simulink model "test_pi_av_formation_event_gazebodirected23a"  (R2023a)
settings: Solver=FixedStepAuto  StartTime=0.0  StopTime=inf  RelTol=1e-3
undefined symbols (not defined in the file or in its folder): angular, DiscIntNeverNeededParam, linear
libraries: ros2lib x28, simulink x8, robotcorelib x8
(part 4 of 4)

== matlab function test_pi_av_formation_event_gazebodirected23a/Translational Control1/Flocking1/MATLAB Function2 ==
  data: ui_prev input; xi input; yi input; zi input; ui_gamma output; xr1 input; yr1 input; zr1 input; xr2 input; yr2 input; zr2 input; xr3 input; yr3 input; zr3 input; iep input size=3; norm_ex input; norm_ey input; norm_ez input; ep output size=3; K_cts input

function [ui_gamma, ep] = naviFeedback(ui_prev, xi, yi, zi, xr1, yr1, zr1, xr2, yr2, zr2, xr3, yr3, zr3, iep, norm_ex, norm_ey, norm_ez, K_cts)
    
    Kpxy = K_cts(1); Kixy = K_cts(2);
    xmin_xy = K_cts(3); xmax_xy = K_cts(4);
    Kpz = K_cts(5); Kiz = K_cts(6);
    xmin_z = K_cts(7); xmax_z = K_cts(8);

    %Sepration control
    ui_xprev = ui_prev(1); ui_yprev = ui_prev(2); ui_zprev = ui_prev(3);

%Errors
    e_x = (xi - xr1 + 0.55) + (xi - xr2) + (xi - xr3 + 1.1);

    e_y = (yi - yr1 + 0.55) + (yi - yr2 + 1.1) + (yi - yr3 + 1.1);

    e_z = (zi - zr1 + 0.55) + (zi - zr2 + 1.1) + (zi - zr3);
       
    ep = [e_x;e_y;e_z];

    if  norm_ex >= 0
        ui_gammax = (-1)* satFcn_esc(Kpxy*e_x, xmin_xy, xmax_xy) + (-1)* satFcn_esc(Kixy*iep(1), xmin_xy, xmax_xy);
    else
        ui_gammax = ui_xprev;
    end

    if  norm_ey >= 0
        ui_gammay = (-1)* satFcn_esc(Kpxy*e_y, xmin_xy, xmax_xy) + (-1)* satFcn_esc(Kixy*iep(1), xmin_xy, xmax_xy);
    else
        ui_gammay = ui_yprev;
    end

    if  norm_ez >= 0
        ui_gammaz = (-1)* satFcn_esc(Kpz*e_z, xmin_z, xmax_z) + (-1)*satFcn_esc(Kiz*iep(3), xmin_z, xmax_z);
    else
        ui_gammaz = ui_zprev;
    end
    

    ui_gamma = [ui_gammax;ui_gammay;ui_gammaz];
    
end

== matlab function test_pi_av_formation_event_gazebodirected23a/Translational Control2/Flocking1/MATLAB Function5 ==
  data: dot_hat_q output; L input; q input; q_hat input; eta1 input; eta2 input; u input; dot_eta output; ddot_eta output
function [dot_hat_q, dot_eta, ddot_eta] = fcn(L, q, q_hat, eta1, eta2, u)

%%separation gains vectors
l2 = [L(1) L(2) L(3)];
l1 = [L(4) L(5) L(6)];
l0 = [L(7) L(8) L(9)];

L_2 = diag(l2);
L_1 = diag(l1);
L_0 = diag(l0);

dot_hat_q = q_est(u, eta1, L_2, q, q_hat);

dot_eta = dot_eta_one(eta2, L_1, q, q_hat);

ddot_eta = dot_eta_two(L_0, q, q_hat);

== matlab function test_pi_av_formation_event_gazebodirected23a/Translational Control3/Flocking1/MATLAB Function5 ==
  data: dot_hat_q output; L input; q input; q_hat input; eta1 input; eta2 input; u input; dot_eta output; ddot_eta output
function [dot_hat_q, dot_eta, ddot_eta] = fcn(L, q, q_hat, eta1, eta2, u)

%%separation gains vectors
l2 = [L(1) L(2) L(3)];
l1 = [L(4) L(5) L(6)];
l0 = [L(7) L(8) L(9)];

L_2 = diag(l2);
L_1 = diag(l1);
L_0 = diag(l0);

dot_hat_q = q_est(u, eta1, L_2, q, q_hat);

dot_eta = dot_eta_one(eta2, L_1, q, q_hat);

ddot_eta = dot_eta_two(L_0, q, q_hat);

== matlab function test_pi_av_formation_event_gazebodirected23a/Translational Control5/Flocking1/MATLAB Function3 ==
  data: ui_prev input; xi input; yi input; zi input; ui_gamma output; xr1 input; yr1 input; zr1 input; xr2 input; yr2 input; zr2 input; iep input size=3; norm_ex input; norm_ey input; norm_ez input; ep output size=3; K_cts input

function [ui_gamma, ep] = naviFeedback(ui_prev, xi, yi, zi, xr1, yr1, zr1, xr2, yr2, zr2, iep, norm_ex, norm_ey, norm_ez, K_cts)
    
    Kpxy = K_cts(1); Kixy = K_cts(2);
    xmin_xy = K_cts(3); xmax_xy = K_cts(4);
    Kpz = K_cts(5); Kiz = K_cts(6);
    xmin_z = K_cts(7); xmax_z = K_cts(8);

    %Sepration control
    ui_xprev = ui_prev(1); ui_yprev = ui_prev(2); ui_zprev = ui_prev(3);

%Errors
    e_x = (xi - xr1 + 0.55) + (xi - xr2 + 1.1);

    e_y = (yi - yr1 + 0.55) + (yi - yr2 + 1.1);

    e_z = (zi - zr1 - 1.1) + (zi - zr2 - 1.1);
       
    ep = [e_x;e_y;e_z];

    if  norm_ex >= 0
        ui_gammax = (-1)* satFcn_esc(Kpxy*e_x, xmin_xy, xmax_xy) + (-1)* satFcn_esc(Kixy*iep(1), xmin_xy, xmax_xy);
    else
        ui_gammax = ui_xprev;
    end

    if  norm_ey >= 0
        ui_gammay = (-1)* satFcn_esc(Kpxy*e_y, xmin_xy, xmax_xy) + (-1)* satFcn_esc(Kixy*iep(1), xmin_xy, xmax_xy);
    else
        ui_gammay = ui_yprev;
    end

    if  norm_ez >= 0
        ui_gammaz = (-1)* satFcn_esc(Kpz*e_z, xmin_z, xmax_z) + (-1)*satFcn_esc(Kiz*iep(3), xmin_z, xmax_z);
    else
        ui_gammaz = ui_zprev;
    end
    

    ui_gamma = [ui_gammax;ui_gammay;ui_gammaz];
    
end

== matlab function test_pi_av_formation_event_gazebodirected23a/Translational Control5/Flocking1/MATLAB Function ==
  data: xi input; yi input; zi input; phiAlpha output; xj input; yj input; zj input; xk input; yk input; zk input; xl input; yl input; zl input; xm input; ym input; zm input; xn input; yn input; zn input; xo input; yo input; zo input; xp input; yp input; zp input; params input

function phiAlpha  = phiAlphaFcn(xi, yi, zi, xj, yj, zj, xk, yk, zk, xl, yl, zl, xm, ym, zm, xn, yn, zn, xo, yo, zo, xp, yp, zp, params)
    
    % Flocking parameters
    epsilon = params(1); a = params(2); b = params(3); c = params(4); d = params(5); h = params(6);

    e = abs(a - b) / sqrt(4*a*b) ;

    cAlpha = sigmaNormFun(c, epsilon) ;
    dAlpha = sigmaNormFun(d, epsilon) ;

    %%
    Pi = [xi;yi;zi] ;

    Pj = [xj;yj;zj] ;
    Pk = [xk;yk;zk] ;
    Pl = [xl;yl;zl] ;
    Pm = [xm;ym;zm] ;
    Pn = [xn;yn;zn] ;
    Po = [xo;yo;zo] ;
    Pp = [xp;yp;zp] ;

    %%
    sigmaNormj = sigmaNormFun(Pj - Pi, epsilon) ;
    nij = gradSigmaFun(Pj - Pi, epsilon) ;
    
    sigmaNormk = sigmaNormFun(Pk - Pi, epsilon) ;
    nik = gradSigmaFun(Pk - Pi, epsilon) ;

    sigmaNorml = sigmaNormFun(Pl - Pi, epsilon) ;
    nil = gradSigmaFun(Pl - Pi, epsilon) ;

    sigmaNormm = sigmaNormFun(Pm - Pi, epsilon) ;
    nim = gradSigmaFun(Pm - Pi, epsilon) ;

    sigmaNormn = sigmaNormFun(Pn - Pi, epsilon) ;
    nin = gradSigmaFun(Pn - Pi, epsilon) ;

    sigmaNormo = sigmaNormFun(Po - Pi, epsilon) ;
    nio = gradSigmaFun(Po - Pi, epsilon) ;

    sigmaNormp = sigmaNormFun(Pp - Pi, epsilon) ;
    nip = gradSigmaFun(Pp - Pi, epsilon) ;

    %%
    sigma1j = sigma1Fun(sigmaNormj - dAlpha + e) ;
    sigma1k = sigma1Fun(sigmaNormk - dAlpha + e) ;
    sigma1l = sigma1Fun(sigmaNorml - dAlpha + e) ;
    sigma1m = sigma1Fun(sigmaNormm - dAlpha + e) ;
    sigma1n = sigma1Fun(sigmaNormn - dAlpha + e) ;
    sigma1o = sigma1Fun(sigmaNormo - dAlpha + e) ;
    sigma1p = sigma1Fun(sigmaNormp - dAlpha + e) ;
            
    %% Position
    phiAlphaj = 0.5 * bumpFcn(sigmaNormj/cAlpha,h) * ((a+b)*sigma1j + (a-b)) ;
    phiAlphanij = phiAlphaj.* nij ;
    
    phiAlphak = 0.5 * bumpFcn(sigmaNormk/cAlpha,h) * ((a+b)*sigma1k + (a-b)) ;
    phiAlphanik = phiAlphak.* nik ;

    phiAlphal = 0.5 * bumpFcn(sigmaNorml/cAlpha,h) * ((a+b)*sigma1l + (a-b)) ;
    phiAlphanil = phiAlphal.* nil ;

    phiAlpham = 0.5 * bumpFcn(sigmaNormm/cAlpha,h) * ((a+b)*sigma1m + (a-b)) ;
    phiAlphanim = phiAlpham.* nim ;

    phiAlphan = 0.5 * bumpFcn(sigmaNormn/cAlpha,h) * ((a+b)*sigma1n + (a-b)) ;
    phiAlphanin = phiAlphan.* nin ;

    phiAlphao = 0.5 * bumpFcn(sigmaNormo/cAlpha,h) * ((a+b)*sigma1o + (a-b)) ;
    phiAlphanio = phiAlphao.* nio ;

    phiAlphap = 0.5 * bumpFcn(sigmaNormp/cAlpha,h) * ((a+b)*sigma1p + (a-b)) ;
    phiAlphanip = phiAlphap.* nip ;


    phiAlpha = phiAlphanij + phiAlphanik + phiAlphanil + phiAlphanim  + phiAlphanin + phiAlphanio + phiAlphanip;

    
end

== matlab function test_pi_av_formation_event_gazebodirected23a/Translational Control5/Flocking1/MATLAB Function1 ==
  data: eta input; phiAlpha input; phiAlpha_int input; ui_gamma input; yaw input; ieyaw input; Ui_pos output size=3; ui_yaw output; KP input; eyaw2 output size=1; eyaw1 input; eyaw2 input; eyaw3 input; eyaw4 input; eyaw6 input; eyaw7 input; eyaw8 input

function [Ui_pos, ui_yaw, eyaw2]  = ctrlLaw(eta, phiAlpha, phiAlpha_int, ui_gamma, yaw, ieyaw, KP, eyaw1, eyaw2, eyaw3, eyaw4, eyaw6, eyaw7, eyaw8)  %, phiBetak, bikobs, phiBetanei, bikve
    
    % Control gains and parameters
    Kx = KP(1); Ky = KP(2); Kz = KP(3);
    Kix = KP(4); Kiy = KP(5); Kiz = KP(6);
    Kyaw = KP(7); Kdyaw = KP(8); Kiyaw = KP(9);
    offset = KP(10);

    eyaw = 0 - yaw(1);
    deyaw = 0 - yaw(2);

    ui_yaw = Kyaw*eyaw + Kdyaw*deyaw + Kiyaw*ieyaw;
    hz_dot = Kz * phiAlpha(3,1) + Kiz * phiAlpha_int(3,1) + ui_gamma(3,1) - eta(3,1);  
    
    if eyaw < offset && eyaw > -offset && eyaw1 < offset && eyaw1 > -offset && eyaw2 < offset && eyaw2 > -offset && eyaw3 < offset && eyaw3 > -offset && eyaw4 < offset && eyaw4 > -offset && eyaw6 < offset && eyaw6 > -offset && eyaw7 < offset && eyaw7 > -offset && eyaw8 < offset && eyaw8 > -offset
        hx_dot = Kx * phiAlpha(1,1) + Kix * phiAlpha_int(1,1) + ui_gamma(1,1) - eta(1,1);  
        hy_dot = Ky * phiAlpha(2,1) + Kiy * phiAlpha_int(2,1) + ui_gamma(2,1) - eta(2,1);  
    else
        hx_dot = 0;
        hy_dot = 0;
    end

    Ui_pos = [hx_dot; hy_dot; hz_dot] ;
    

end

== matlab function test_pi_av_formation_event_gazebodirected23a/Translational Control6/Flocking1/MATLAB Function3 ==
  data: ui_prev input; xi input; yi input; zi input; ui_gamma output; xr1 input; yr1 input; zr1 input; xr2 input; yr2 input; zr2 input; xr3 input; yr3 input; zr3 input; iep input size=3; norm_ex input; norm_ey input; norm_ez input; ep output size=3; K_cts input

function [ui_gamma, ep] = naviFeedback(ui_prev, xi, yi, zi, xr1, yr1, zr1, xr2, yr2, zr2, xr3, yr3, zr3, iep, norm_ex, norm_ey, norm_ez, K_cts)
    
    Kpxy = K_cts(1); Kixy = K_cts(2);
    xmin_xy = K_cts(3); xmax_xy = K_cts(4);
    Kpz = K_cts(5); Kiz = K_cts(6);
    xmin_z = K_cts(7); xmax_z = K_cts(8);

    %Sepration control
    ui_xprev = ui_prev(1); ui_yprev = ui_prev(2); ui_zprev = ui_prev(3);

%Errors
    e_x = (xi - xr1 - 0.55) + (xi - xr2) + (xi - xr3 - 1.1);

    e_y = (yi - yr1 + 0.55) + (yi - yr2 + 1.1) + (yi - yr3);

    e_z = (zi - zr1 - 0.55) + (zi - zr2 - 1.1) + (zi - zr3);
       
    ep = [e_x;e_y;e_z];

    if  norm_ex >= 0
        ui_gammax = (-1)* satFcn_esc(Kpxy*e_x, xmin_xy, xmax_xy) + (-1)* satFcn_esc(Kixy*iep(1), xmin_xy, xmax_xy);
    else
        ui_gammax = ui_xprev;
    end

    if  norm_ey >= 0
        ui_gammay = (-1)* satFcn_esc(Kpxy*e_y, xmin_xy, xmax_xy) + (-1)* satFcn_esc(Kixy*iep(1), xmin_xy, xmax_xy);
    else
        ui_gammay = ui_yprev;
    end

    if  norm_ez >= 0
        ui_gammaz = (-1)* satFcn_esc(Kpz*e_z, xmin_z, xmax_z) + (-1)*satFcn_esc(Kiz*iep(3), xmin_z, xmax_z);
    else
        ui_gammaz = ui_zprev;
    end
    

    ui_gamma = [ui_gammax;ui_gammay;ui_gammaz];
    
end

== matlab function test_pi_av_formation_event_gazebodirected23a/Translational Control5/Flocking1/MATLAB Function5 ==
  data: dot_hat_q output; L input; q input; q_hat input; eta1 input; eta2 input; u input; dot_eta output; ddot_eta output
function [dot_hat_q, dot_eta, ddot_eta] = fcn(L, q, q_hat, eta1, eta2, u)

%%separation gains vectors
l2 = [L(1) L(2) L(3)];
l1 = [L(4) L(5) L(6)];
l0 = [L(7) L(8) L(9)];

L_2 = diag(l2);
L_1 = diag(l1);
L_0 = diag(l0);

dot_hat_q = q_est(u, eta1, L_2, q, q_hat);

dot_eta = dot_eta_one(eta2, L_1, q, q_hat);

ddot_eta = dot_eta_two(L_0, q, q_hat);

== matlab function test_pi_av_formation_event_gazebodirected23a/Translational Control7/Flocking1/MATLAB Function ==
  data: xi input; yi input; zi input; phiAlpha output; xj input; yj input; zj input; xk input; yk input; zk input; xl input; yl input; zl input; xm input; ym input; zm input; xn input; yn input; zn input; xo input; yo input; zo input; xp input; yp input; zp input; params input

function phiAlpha  = phiAlphaFcn(xi, yi, zi, xj, yj, zj, xk, yk, zk, xl, yl, zl, xm, ym, zm, xn, yn, zn, xo, yo, zo, xp, yp, zp, params)
    
    % Flocking parameters
    epsilon = params(1); a = params(2); b = params(3); c = params(4); d = params(5); h = params(6);

    e = abs(a - b) / sqrt(4*a*b) ;

    cAlpha = sigmaNormFun(c, epsilon) ;
    dAlpha = sigmaNormFun(d, epsilon) ;

    %%
    Pi = [xi;yi;zi] ;

    Pj = [xj;yj;zj] ;
    Pk = [xk;yk;zk] ;
    Pl = [xl;yl;zl] ;
    Pm = [xm;ym;zm] ;
    Pn = [xn;yn;zn] ;
    Po = [xo;yo;zo] ;
    Pp = [xp;yp;zp] ;

    %%
    sigmaNormj = sigmaNormFun(Pj - Pi, epsilon) ;
    nij = gradSigmaFun(Pj - Pi, epsilon) ;
    
    sigmaNormk = sigmaNormFun(Pk - Pi, epsilon) ;
    nik = gradSigmaFun(Pk - Pi, epsilon) ;

    sigmaNorml = sigmaNormFun(Pl - Pi, epsilon) ;
    nil = gradSigmaFun(Pl - Pi, epsilon) ;

    sigmaNormm = sigmaNormFun(Pm - Pi, epsilon) ;
    nim = gradSigmaFun(Pm - Pi, epsilon) ;

    sigmaNormn = sigmaNormFun(Pn - Pi, epsilon) ;
    nin = gradSigmaFun(Pn - Pi, epsilon) ;

    sigmaNormo = sigmaNormFun(Po - Pi, epsilon) ;
    nio = gradSigmaFun(Po - Pi, epsilon) ;

    sigmaNormp = sigmaNormFun(Pp - Pi, epsilon) ;
    nip = gradSigmaFun(Pp - Pi, epsilon) ;

    %%
    sigma1j = sigma1Fun(sigmaNormj - dAlpha + e) ;
    sigma1k = sigma1Fun(sigmaNormk - dAlpha + e) ;
    sigma1l = sigma1Fun(sigmaNorml - dAlpha + e) ;
    sigma1m = sigma1Fun(sigmaNormm - dAlpha + e) ;
    sigma1n = sigma1Fun(sigmaNormn - dAlpha + e) ;
    sigma1o = sigma1Fun(sigmaNormo - dAlpha + e) ;
    sigma1p = sigma1Fun(sigmaNormp - dAlpha + e) ;
            
    %% Position
    phiAlphaj = 0.5 * bumpFcn(sigmaNormj/cAlpha,h) * ((a+b)*sigma1j + (a-b)) ;
    phiAlphanij = phiAlphaj.* nij ;
    
    phiAlphak = 0.5 * bumpFcn(sigmaNormk/cAlpha,h) * ((a+b)*sigma1k + (a-b)) ;
    phiAlphanik = phiAlphak.* nik ;

    phiAlphal = 0.5 * bumpFcn(sigmaNorml/cAlpha,h) * ((a+b)*sigma1l + (a-b)) ;
    phiAlphanil = phiAlphal.* nil ;

    phiAlpham = 0.5 * bumpFcn(sigmaNormm/cAlpha,h) * ((a+b)*sigma1m + (a-b)) ;
    phiAlphanim = phiAlpham.* nim ;

    phiAlphan = 0.5 * bumpFcn(sigmaNormn/cAlpha,h) * ((a+b)*sigma1n + (a-b)) ;
    phiAlphanin = phiAlphan.* nin ;

    phiAlphao = 0.5 * bumpFcn(sigmaNormo/cAlpha,h) * ((a+b)*sigma1o + (a-b)) ;
    phiAlphanio = phiAlphao.* nio ;

    phiAlphap = 0.5 * bumpFcn(sigmaNormp/cAlpha,h) * ((a+b)*sigma1p + (a-b)) ;
    phiAlphanip = phiAlphap.* nip ;


    phiAlpha = phiAlphanij + phiAlphanik + phiAlphanil + phiAlphanim  + phiAlphanin + phiAlphanio + phiAlphanip;

    
end

== matlab function test_pi_av_formation_event_gazebodirected23a/Translational Control7/Flocking1/MATLAB Function1 ==
  data: eta input; phiAlpha input; phiAlpha_int input; ui_gamma input; yaw input; ieyaw input; Ui_pos output size=3; ui_yaw output; KP input; eyaw2 output size=1; eyaw1 input; eyaw2 input; eyaw3 input; eyaw4 input; eyaw5 input; eyaw6 input; eyaw8 input

function [Ui_pos, ui_yaw, eyaw2]  = ctrlLaw(eta, phiAlpha, phiAlpha_int, ui_gamma, yaw, ieyaw, KP, eyaw1, eyaw2, eyaw3, eyaw4, eyaw5, eyaw6, eyaw8)  %, phiBetak, bikobs, phiBetanei, bikve
    
    % Control gains and parameters
    Kx = KP(1); Ky = KP(2); Kz = KP(3);
    Kix = KP(4); Kiy = KP(5); Kiz = KP(6);
    Kyaw = KP(7); Kdyaw = KP(8); Kiyaw = KP(9);
    offset = KP(10);

    eyaw = 0 - yaw(1);
    deyaw = 0 - yaw(2);

    ui_yaw = Kyaw*eyaw + Kdyaw*deyaw + Kiyaw*ieyaw;
    hz_dot = Kz * phiAlpha(3,1) + Kiz * phiAlpha_int(3,1) + ui_gamma(3,1) - eta(3,1);  
    
    if eyaw < offset && eyaw > -offset && eyaw1 < offset && eyaw1 > -offset && eyaw2 < offset && eyaw2 > -offset && eyaw3 < offset && eyaw3 > -offset && eyaw4 < offset && eyaw4 > -offset && eyaw5 < offset && eyaw5 > -offset && eyaw6 < offset && eyaw6 > -offset && eyaw8 < offset && eyaw8 > -offset
        hx_dot = Kx * phiAlpha(1,1) + Kix * phiAlpha_int(1,1) + ui_gamma(1,1) - eta(1,1);  
        hy_dot = Ky * phiAlpha(2,1) + Kiy * phiAlpha_int(2,1) + ui_gamma(2,1) - eta(2,1);  
    else
        hx_dot = 0;
        hy_dot = 0;
    end

    Ui_pos = [hx_dot; hy_dot; hz_dot] ;
    

end

== matlab function test_pi_av_formation_event_gazebodirected23a/Translational Control8/Flocking1/MATLAB Function3 ==
  data: ui_prev input; xi input; yi input; zi input; ui_gamma output; xr1 input; yr1 input; zr1 input; xr2 input; yr2 input; zr2 input; xr3 input; yr3 input; zr3 input; iep input size=3; norm_ex input; norm_ey input; norm_ez input; ep output size=3; K_cts input

function [ui_gamma, ep] = naviFeedback(ui_prev, xi, yi, zi, xr1, yr1, zr1, xr2, yr2, zr2, xr3, yr3, zr3, iep, norm_ex, norm_ey, norm_ez, K_cts)
    
    Kpxy = K_cts(1); Kixy = K_cts(2);
    xmin_xy = K_cts(3); xmax_xy = K_cts(4);
    Kpz = K_cts(5); Kiz = K_cts(6);
    xmin_z = K_cts(7); xmax_z = K_cts(8);

    %Sepration control
    ui_xprev = ui_prev(1); ui_yprev = ui_prev(2); ui_zprev = ui_prev(3);

%Errors
    e_x = (xi - xr1 + 0.55) + (xi - xr2)  + (xi - xr3 + 1.1);

    e_y = (yi - yr1 - 0.55) + (yi - yr2 - 1.1) + (yi - yr3);

    e_z = (zi - zr1 - 0.55) + (zi - zr2 - 1.1) + (zi - zr3 - 1.1);
       
    ep = [e_x;e_y;e_z];

    if  norm_ex >= 0
        ui_gammax = (-1)* satFcn_esc(Kpxy*e_x, xmin_xy, xmax_xy) + (-1)* satFcn_esc(Kixy*iep(1), xmin_xy, xmax_xy);
    else
        ui_gammax = ui_xprev;
    end

    if  norm_ey >= 0
        ui_gammay = (-1)* satFcn_esc(Kpxy*e_y, xmin_xy, xmax_xy) + (-1)* satFcn_esc(Kixy*iep(1), xmin_xy, xmax_xy);
    else
        ui_gammay = ui_yprev;
    end

    if  norm_ez >= 0
        ui_gammaz = (-1)* satFcn_esc(Kpz*e_z, xmin_z, xmax_z) + (-1)*satFcn_esc(Kiz*iep(3), xmin_z, xmax_z);
    else
        ui_gammaz = ui_zprev;
    end
    

    ui_gamma = [ui_gammax;ui_gammay;ui_gammaz];
    
end

== matlab function test_pi_av_formation_event_gazebodirected23a/Translational Control1/Flocking1/MATLAB Function5 ==
  data: dot_hat_q output; L input; q input; q_hat input; eta1 input; eta2 input; u input; dot_eta output; ddot_eta output
function [dot_hat_q, dot_eta, ddot_eta] = fcn(L, q, q_hat, eta1, eta2, u)

%%separation gains vectors
l2 = [L(1) L(2) L(3)];
l1 = [L(4) L(5) L(6)];
l0 = [L(7) L(8) L(9)];

L_2 = diag(l2);
L_1 = diag(l1);
L_0 = diag(l0);

dot_hat_q = q_est(u, eta1, L_2, q, q_hat);

dot_eta = dot_eta_one(eta2, L_1, q, q_hat);

ddot_eta = dot_eta_two(L_0, q, q_hat);

== matlab function test_pi_av_formation_event_gazebodirected23a/Translational Control7/Flocking1/MATLAB Function5 ==
  data: dot_hat_q output; L input; q input; q_hat input; eta1 input; eta2 input; u input; dot_eta output; ddot_eta output
function [dot_hat_q, dot_eta, ddot_eta] = fcn(L, q, q_hat, eta1, eta2, u)

%%separation gains vectors
l2 = [L(1) L(2) L(3)];
l1 = [L(4) L(5) L(6)];
l0 = [L(7) L(8) L(9)];

L_2 = diag(l2);
L_1 = diag(l1);
L_0 = diag(l0);

dot_hat_q = q_est(u, eta1, L_2, q, q_hat);

dot_eta = dot_eta_one(eta2, L_1, q, q_hat);

ddot_eta = dot_eta_two(L_0, q, q_hat);

== matlab function test_pi_av_formation_event_gazebodirected23a/Translational Control8/Flocking1/MATLAB Function ==
  data: xi input; yi input; zi input; phiAlpha output; xj input; yj input; zj input; xk input; yk input; zk input; xl input; yl input; zl input; xm input; ym input; zm input; xn input; yn input; zn input; xo input; yo input; zo input; xp input; yp input; zp input; params input

function phiAlpha  = phiAlphaFcn(xi, yi, zi, xj, yj, zj, xk, yk, zk, xl, yl, zl, xm, ym, zm, xn, yn, zn, xo, yo, zo, xp, yp, zp, params)
    
    % Flocking parameters
    epsilon = params(1); a = params(2); b = params(3); c = params(4); d = params(5); h = params(6);

    e = abs(a - b) / sqrt(4*a*b) ;

    cAlpha = sigmaNormFun(c, epsilon) ;
    dAlpha = sigmaNormFun(d, epsilon) ;

    %%
    Pi = [xi;yi;zi] ;

    Pj = [xj;yj;zj] ;
    Pk = [xk;yk;zk] ;
    Pl = [xl;yl;zl] ;
    Pm = [xm;ym;zm] ;
    Pn = [xn;yn;zn] ;
    Po = [xo;yo;zo] ;
    Pp = [xp;yp;zp] ;

    %%
    sigmaNormj = sigmaNormFun(Pj - Pi, epsilon) ;
    nij = gradSigmaFun(Pj - Pi, epsilon) ;
    
    sigmaNormk = sigmaNormFun(Pk - Pi, epsilon) ;
    nik = gradSigmaFun(Pk - Pi, epsilon) ;

    sigmaNorml = sigmaNormFun(Pl - Pi, epsilon) ;
    nil = gradSigmaFun(Pl - Pi, epsilon) ;

    sigmaNormm = sigmaNormFun(Pm - Pi, epsilon) ;
    nim = gradSigmaFun(Pm - Pi, epsilon) ;

    sigmaNormn = sigmaNormFun(Pn - Pi, epsilon) ;
    nin = gradSigmaFun(Pn - Pi, epsilon) ;

    sigmaNormo = sigmaNormFun(Po - Pi, epsilon) ;
    nio = gradSigmaFun(Po - Pi, epsilon) ;

    sigmaNormp = sigmaNormFun(Pp - Pi, epsilon) ;
    nip = gradSigmaFun(Pp - Pi, epsilon) ;

    %%
    sigma1j = sigma1Fun(sigmaNormj - dAlpha + e) ;
    sigma1k = sigma1Fun(sigmaNormk - dAlpha + e) ;
    sigma1l = sigma1Fun(sigmaNorml - dAlpha + e) ;
    sigma1m = sigma1Fun(sigmaNormm - dAlpha + e) ;
    sigma1n = sigma1Fun(sigmaNormn - dAlpha + e) ;
    sigma1o = sigma1Fun(sigmaNormo - dAlpha + e) ;
    sigma1p = sigma1Fun(sigmaNormp - dAlpha + e) ;
            
    %% Position
    phiAlphaj = 0.5 * bumpFcn(sigmaNormj/cAlpha,h) * ((a+b)*sigma1j + (a-b)) ;
    phiAlphanij = phiAlphaj.* nij ;
    
    phiAlphak = 0.5 * bumpFcn(sigmaNormk/cAlpha,h) * ((a+b)*sigma1k + (a-b)) ;
    phiAlphanik = phiAlphak.* nik ;

    phiAlphal = 0.5 * bumpFcn(sigmaNorml/cAlpha,h) * ((a+b)*sigma1l + (a-b)) ;
    phiAlphanil = phiAlphal.* nil ;

    phiAlpham = 0.5 * bumpFcn(sigmaNormm/cAlpha,h) * ((a+b)*sigma1m + (a-b)) ;
    phiAlphanim = phiAlpham.* nim ;

    phiAlphan = 0.5 * bumpFcn(sigmaNormn/cAlpha,h) * ((a+b)*sigma1n + (a-b)) ;
    phiAlphanin = phiAlphan.* nin ;

    phiAlphao = 0.5 * bumpFcn(sigmaNormo/cAlpha,h) * ((a+b)*sigma1o + (a-b)) ;
    phiAlphanio = phiAlphao.* nio ;

    phiAlphap = 0.5 * bumpFcn(sigmaNormp/cAlpha,h) * ((a+b)*sigma1p + (a-b)) ;
    phiAlphanip = phiAlphap.* nip ;


    phiAlpha = phiAlphanij + phiAlphanik + phiAlphanil + phiAlphanim  + phiAlphanin + phiAlphanio + phiAlphanip;

    
end

== matlab function test_pi_av_formation_event_gazebodirected23a/Translational Control4/Flocking1/MATLAB Function5 ==
  data: dot_hat_q output; L input; q input; q_hat input; eta1 input; eta2 input; u input; dot_eta output; ddot_eta output
function [dot_hat_q, dot_eta, ddot_eta] = fcn(L, q, q_hat, eta1, eta2, u)

%%separation gains vectors
l2 = [L(1) L(2) L(3)];
l1 = [L(4) L(5) L(6)];
l0 = [L(7) L(8) L(9)];

L_2 = diag(l2);
L_1 = diag(l1);
L_0 = diag(l0);

dot_hat_q = q_est(u, eta1, L_2, q, q_hat);

dot_eta = dot_eta_one(eta2, L_1, q, q_hat);

ddot_eta = dot_eta_two(L_0, q, q_hat);

== matlab function test_pi_av_formation_event_gazebodirected23a/Translational Control8/Flocking1/MATLAB Function1 ==
  data: eta input; phiAlpha input; phiAlpha_int input; ui_gamma input; yaw input; ieyaw input; Ui_pos output size=3; ui_yaw output; KP input; eyaw2 output size=1; eyaw1 input; eyaw2 input; eyaw3 input; eyaw4 input; eyaw5 input; eyaw6 input; eyaw7 input

function [Ui_pos, ui_yaw, eyaw2]  = ctrlLaw(eta, phiAlpha, phiAlpha_int, ui_gamma, yaw, ieyaw, KP, eyaw1, eyaw2, eyaw3, eyaw4, eyaw5, eyaw6, eyaw7)  %, phiBetak, bikobs, phiBetanei, bikve
    
    % Control gains and parameters
    Kx = KP(1); Ky = KP(2); Kz = KP(3);
    Kix = KP(4); Kiy = KP(5); Kiz = KP(6);
    Kyaw = KP(7); Kdyaw = KP(8); Kiyaw = KP(9);
    offset = KP(10);

    eyaw = 0 - yaw(1);
    deyaw = 0 - yaw(2);

    ui_yaw = Kyaw*eyaw + Kdyaw*deyaw + Kiyaw*ieyaw;
    hz_dot = Kz * phiAlpha(3,1) + Kiz * phiAlpha_int(3,1) + ui_gamma(3,1) - eta(3,1);  
    
    if eyaw < offset && eyaw > -offset && eyaw1 < offset && eyaw1 > -offset && eyaw2 < offset && eyaw2 > -offset && eyaw3 < offset && eyaw3 > -offset && eyaw4 < offset && eyaw4 > -offset && eyaw5 < offset && eyaw5 > -offset && eyaw6 < offset && eyaw6 > -offset && eyaw7 < offset && eyaw7 > -offset
        hx_dot = Kx * phiAlpha(1,1) + Kix * phiAlpha_int(1,1) + ui_gamma(1,1) - eta(1,1);  
        hy_dot = Ky * phiAlpha(2,1) + Kiy * phiAlpha_int(2,1) + ui_gamma(2,1) - eta(2,1);  
    else
        hx_dot = 0;
        hy_dot = 0;
    end

    Ui_pos = [hx_dot; hy_dot; hz_dot] ;
    

end

== matlab function test_pi_av_formation_event_gazebodirected23a/Translational Control1/Flocking1/event_x2 ==
  data: e_1 output; e_2 output; e1 input; e2 input; e3 input; e_3 output; i1 output; i1 input; i2 input; i3 input; i2 output; i3 output
function [e_1,e_2, e_3, i1, i2, i3]  = fcn(e1, e2, e3, i1, i2, i3)

if e1 >= 0
    e_1 = 1;
    i1 = i1+1;
else 
    e_1 = 0;
    i1 = i1;
end

if e2 >= 0
    e_2 = 1;
    i2 = i2 + 1;
else 
    e_2 = 0;
    i2 = i2;
end

if e3 >= 0
    e_3 = 1;
    i3 = i3 + 1;
else 
    e_3 = 0;
    i3 = i3;
end

== matlab function test_pi_av_formation_event_gazebodirected23a/Translational Control8/Flocking1/MATLAB Function5 ==
  data: dot_hat_q output; L input; q input; q_hat input; eta1 input; eta2 input; u input; dot_eta output; ddot_eta output
function [dot_hat_q, dot_eta, ddot_eta] = fcn(L, q, q_hat, eta1, eta2, u)

%%separation gains vectors
l2 = [L(1) L(2) L(3)];
l1 = [L(4) L(5) L(6)];
l0 = [L(7) L(8) L(9)];

L_2 = diag(l2);
L_1 = diag(l1);
L_0 = diag(l0);

dot_hat_q = q_est(u, eta1, L_2, q, q_hat);

dot_eta = dot_eta_one(eta2, L_1, q, q_hat);

ddot_eta = dot_eta_two(L_0, q, q_hat);

== matlab function test_pi_av_formation_event_gazebodirected23a/MATLAB Function2 ==
  data: data input; y output
function y = fcn(data)

DATA = data(1:20);
d1 = awgn(double(DATA(1)), 33, 'measured');
d2 = awgn(double(DATA(2)), 33, 'measured');
d3 = awgn(double(DATA(3)), 33, 'measured');
d4 = awgn(double(DATA(4)), 33, 'measured');
d5 = awgn(double(DATA(5)), 33, 'measured');
d6 = awgn(double(DATA(6)), 33, 'measured');
d7 = awgn(double(DATA(7)), 33, 'measured');
y = [d1;d2;d3;d4;d5;d6;d7];

== matlab function test_pi_av_formation_event_gazebodirected23a/Subsystem1/MATLAB Function6 ==
  data: X1 input; X2 input; X3 input; X4 input; X5 input; X6 input; X7 input; d_meas input; xyz output
function xyz = fcn(X1, X2, X3, X4, X5, X6, X7, d_meas)

%% Extract data from vectors
states1 = X1(1:3);
x1 = states1(1);
y1 = states1(2);
z1 = states1(3);

states2 = X2(1:3);
x2 = states2(1);
y2 = states2(2);
z2 = states2(3);

states3 = X3(1:3);
x3 = states3(1);
y3 = states3(2);
z3 = states3(3);

states4 = X4(1:3);
x4 = states4(1);
y4 = states4(2);
z4 = states4(3);

states5 = X5(1:3);
x5 = states5(1);
y5 = states5(2);
z5 = states5(3);

states6 = X6(1:3);
x6 = states6(1);
y6 = states6(2);
z6 = states6(3);

states7 = X7(1:3);
x7 = states7(1);
y7 = states7(2);
z7 = states7(3);

r1 = d_meas(1);
r2 = d_meas(2);
r3 = d_meas(3);
r4 = d_meas(4);
r5 = d_meas(5);
r6 = d_meas(6);
r7 = d_meas(7);

xyz = multi_fun2(x1, y1, z1, r1, x2, y2, z2, r2, x3, y3, z3, r3, x4, y4, z4, r4, x5, y5, z5, r5, x6, y6, z6, r6, x7, y7, z7, r7);

== matlab function test_pi_av_formation_event_gazebodirected23a/Subsystem1/dist_AVT ==
  data: meas input; u_B input; dU output; dAVT output; avt_pars input
function [dU,dAVT]  = fcn(meas, u_B, avt_pars)

%Vector separation
d1 = meas(1);
d2 = meas(2);
d3 = meas(3);
d4 = meas(4);
d5 = meas(5);
d6 = meas(6);
d7 = meas(7);

avtpars = avt_pars(1:4);
inc = avtpars(1);
dec = avtpars(2);
min = avtpars(3);
max = avtpars(4);

%% memory variables
d_avt1 = u_B(1);
adjustment1 = u_B(2);
s_adjust1 = u_B(3);

d_avt2 = u_B(4);
adjustment2 = u_B(5);
s_adjust2 = u_B(6);

d_avt3 = u_B(7);
adjustment3 = u_B(8);
s_adjust3 = u_B(9);

d_avt4 = u_B(10);
adjustment4 = u_B(11);
s_adjust4 = u_B(12);

d_avt5 = u_B(13);
adjustment5 = u_B(14);
s_adjust5 = u_B(15);

d_avt6 = u_B(16);
adjustment6 = u_B(17);
s_adjust6 = u_B(18);

d_avt7 = u_B(19);
adjustment7 = u_B(20);
s_adjust7 = u_B(21);

%%
du1 = AVTfun(d_avt1, d1, adjustment1, s_adjust1, min, max, inc, dec);

du2 = AVTfun(d_avt2, d2, adjustment2, s_adjust2, min, max, inc, dec);

du3 = AVTfun(d_avt3, d3, adjustment3, s_adjust3, min, max, inc, dec);

du4 = AVTfun(d_avt4, d4, adjustment4, s_adjust4, min, max, inc, dec);

du5 = AVTfun(d_avt5, d5, adjustment5, s_adjust5, min, max, inc, dec);

du6 = AVTfun(d_avt6, d6, adjustment6, s_adjust6, min, max, inc, dec);

du7 = AVTfun(d_avt7, d7, adjustment7, s_adjust7, min, max, inc, dec);

dU = [du1;du2;du3;du4;du5;du6;du7];
dAVT = [du1(1);du2(1);du3(1);du4(1);du5(1);du6(1);du7(1)];

== matlab function test_pi_av_formation_event_gazebodirected23a/MATLAB Function3 ==
  data: data input; y output
function y = fcn(data)

DATA = data(1:20);
d1 = awgn(double(DATA(1)), 33, 'measured');
d2 = awgn(double(DATA(2)), 33, 'measured');
d3 = awgn(double(DATA(3)), 33, 'measured');
d4 = awgn(double(DATA(4)), 33, 'measured');
d5 = awgn(double(DATA(5)), 33, 'measured');
d6 = awgn(double(DATA(6)), 33, 'measured');
d7 = awgn(double(DATA(7)), 33, 'measured');
y = [d1;d2;d3;d4;d5;d6;d7];

== matlab function test_pi_av_formation_event_gazebodirected23a/Subsystem2/MATLAB Function6 ==
  data: X1 input; X2 input; X3 input; X4 input; X5 input; X6 input; X7 input; d_meas input; xyz output
function xyz = fcn(X1, X2, X3, X4, X5, X6, X7, d_meas)

%% Extract data from vectors
states1 = X1(1:3);
x1 = states1(1);
y1 = states1(2);
z1 = states1(3);

states2 = X2(1:3);
x2 = states2(1);
y2 = states2(2);
z2 = states2(3);

states3 = X3(1:3);
x3 = states3(1);
y3 = states3(2);
z3 = states3(3);

states4 = X4(1:3);
x4 = states4(1);
y4 = states4(2);
z4 = states4(3);

states5 = X5(1:3);
x5 = states5(1);
y5 = states5(2);
z5 = states5(3);

states6 = X6(1:3);
x6 = states6(1);
y6 = states6(2);
z6 = states6(3);

states7 = X7(1:3);
x7 = states7(1);
y7 = states7(2);
z7 = states7(3);

r1 = d_meas(1);
r2 = d_meas(2);
r3 = d_meas(3);
r4 = d_meas(4);
r5 = d_meas(5);
r6 = d_meas(6);
r7 = d_meas(7);

xyz = multi_fun2(x1, y1, z1, r1, x2, y2, z2, r2, x3, y3, z3, r3, x4, y4, z4, r4, x5, y5, z5, r5, x6, y6, z6, r6, x7, y7, z7, r7);

== matlab function test_pi_av_formation_event_gazebodirected23a/Subsystem2/dist_AVT ==
  data: meas input; u_B input; dU output; dAVT output; avt_pars input
function [dU,dAVT]  = fcn(meas, u_B, avt_pars)

%Vector separation
d1 = meas(1);
d2 = meas(2);
d3 = meas(3);
d4 = meas(4);
d5 = meas(5);
d6 = meas(6);
d7 = meas(7);

avtpars = avt_pars(1:4);
inc = avtpars(1);
dec = avtpars(2);
min = avtpars(3);
max = avtpars(4);

%% memory variables
d_avt1 = u_B(1);
adjustment1 = u_B(2);
s_adjust1 = u_B(3);

d_avt2 = u_B(4);
adjustment2 = u_B(5);
s_adjust2 = u_B(6);

d_avt3 = u_B(7);
adjustment3 = u_B(8);
s_adjust3 = u_B(9);

d_avt4 = u_B(10);
adjustment4 = u_B(11);
s_adjust4 = u_B(12);

d_avt5 = u_B(13);
adjustment5 = u_B(14);
s_adjust5 = u_B(15);

d_avt6 = u_B(16);
adjustment6 = u_B(17);
s_adjust6 = u_B(18);

d_avt7 = u_B(19);
adjustment7 = u_B(20);
s_adjust7 = u_B(21);

%%
du1 = AVTfun(d_avt1, d1, adjustment1, s_adjust1, min, max, inc, dec);

du2 = AVTfun(d_avt2, d2, adjustment2, s_adjust2, min, max, inc, dec);

du3 = AVTfun(d_avt3, d3, adjustment3, s_adjust3, min, max, inc, dec);

du4 = AVTfun(d_avt4, d4, adjustment4, s_adjust4, min, max, inc, dec);

du5 = AVTfun(d_avt5, d5, adjustment5, s_adjust5, min, max, inc, dec);

du6 = AVTfun(d_avt6, d6, adjustment6, s_adjust6, min, max, inc, dec);

du7 = AVTfun(d_avt7, d7, adjustment7, s_adjust7, min, max, inc, dec);

dU = [du1;du2;du3;du4;du5;du6;du7];
dAVT = [du1(1);du2(1);du3(1);du4(1);du5(1);du6(1);du7(1)];

== matlab function test_pi_av_formation_event_gazebodirected23a/MATLAB Function4 ==
  data: t input; D output
function D = fcn(t)

if t <= 150
    d1 = 0;
    d2 = 0;
    d3 = 0;
else
    d1 = 0.5 + 0.2*sin(t)*0.5*cos(0.1*t) ;
    d2 = -0.4 + 0.2*cos(0.5*t)*cos(0.2*t);
    d3 = 0.01*sin(0.1*t);
end

D = [d1;d2;d3];

== matlab function test_pi_av_formation_event_gazebodirected23a/Translational Control1/Flocking1/event_1 ==
  data: x input; y input; z input; mx input; my input; mz input; norm_ex output; norm_ey output; c0 input; norm_ez output
function [norm_ex, norm_ey, norm_ez] = fcn(x, y, z, mx, my, mz, c0)

cx = c0(1); cy = c0(2); cz = c0(3); 

norm_ex = abs((mx-x)) - cx;
norm_ey = abs((my-y)) - cy;
norm_ez = abs((mz-z)) - cz;

== matlab function test_pi_av_formation_event_gazebodirected23a/Translational Control1/Flocking1/memory_1 ==
  data: ex input; ey input; mx output; ez input; x input; y input; z input; mx input; my input; mz input; my output; mz output
function [mx, my, mz] = fcn(ex, ey, ez, x, y, z, mx, my, mz)

if ex >= 0
    mx = x;    
else
    mx = mx;
end

if ey >= 0
    my = y;    
else
    my = my;
end

if ez >= 0
    mz = z;    
else
    mz = mz;
end

== matlab function test_pi_av_formation_event_gazebodirected23a/Translational Control2/Flocking1/MATLAB Function3 ==
  data: ui_prev input; xi input; yi input; zi input; ui_gamma output; xr1 input; yr1 input; zr1 input; xr2 input; yr2 input; zr2 input; iep input size=3; norm_ex input; norm_ey input; norm_ez input; ep output size=3; K_cts input

function [ui_gamma, ep] = naviFeedback(ui_prev, xi, yi, zi, xr1, yr1, zr1, xr2, yr2, zr2, iep, norm_ex, norm_ey, norm_ez, K_cts)
    
    Kpxy = K_cts(1); Kixy = K_cts(2);
    xmin_xy = K_cts(3); xmax_xy = K_cts(4);
    Kpz = K_cts(5); Kiz = K_cts(6);
    xmin_z = K_cts(7); xmax_z = K_cts(8);

    %Sepration control
    ui_xprev = ui_prev(1); ui_yprev = ui_prev(2); ui_zprev = ui_prev(3);

%Errors
    e_x = (xi - xr1 - 0.55) + (xi - xr2 - 1.1);

    e_y = (yi - yr1 + 0.55) + (yi - yr2);

    e_z = (zi - zr1 + 0.55) + (zi - zr2 + 1.1);
       
    ep = [e_x;e_y;e_z];

    if  norm_ex >= 0
        ui_gammax = (-1)* satFcn_esc(Kpxy*e_x, xmin_xy, xmax_xy) + (-1)* satFcn_esc(Kixy*iep(1), xmin_xy, xmax_xy);
    else
        ui_gammax = ui_xprev;
    end

    if  norm_ey >= 0
        ui_gammay = (-1)* satFcn_esc(Kpxy*e_y, xmin_xy, xmax_xy) + (-1)* satFcn_esc(Kixy*iep(1), xmin_xy, xmax_xy);
    else
        ui_gammay = ui_yprev;
    end

    if  norm_ez >= 0
        ui_gammaz = (-1)* satFcn_esc(Kpz*e_z, xmin_z, xmax_z) + (-1)*satFcn_esc(Kiz*iep(3), xmin_z, xmax_z);
    else
        ui_gammaz = ui_zprev;
    end
    

    ui_gamma = [ui_gammax;ui_gammay;ui_gammaz];
    
end

== matlab function test_pi_av_formation_event_gazebodirected23a/Translational Control2/Flocking1/event_1 ==
  data: x input; y input; z input; mx input; my input; mz input; norm_ex output; norm_ey output; c0 input; norm_ez output
function [norm_ex, norm_ey, norm_ez] = fcn(x, y, z, mx, my, mz, c0)

cx = c0(1); cy = c0(2); cz = c0(3); 

norm_ex = abs((mx-x)) - cx;
norm_ey = abs((my-y)) - cy;
norm_ez = abs((mz-z)) - cz;

== matlab function test_pi_av_formation_event_gazebodirected23a/Translational Control2/Flocking1/memory_1 ==
  data: ex input; ey input; mx output; ez input; x input; y input; z input; mx input; my input; mz input; my output; mz output
function [mx, my, mz] = fcn(ex, ey, ez, x, y, z, mx, my, mz)

if ex >= 0
    mx = x;    
else
    mx = mx;
end

if ey >= 0
    my = y;    
else
    my = my;
end

if ez >= 0
    mz = z;    
else
    mz = mz;
end
